simulink model "main_adaptive"  (R2021b)
settings: Solver=ode45  StartTime=0.0  StopTime=80  FixedStep=0.1  RelTol=1e-4
libraries: slpidlib x6
(part 2 of 2)

== matlab function main_adaptive/Subsystem3/u3 sign 2 ==
  data: y_t input; y_t_1 input; u2_sign output; u2_dis input; u2_dis_t_1 input
function u2_sign  = u2_sing(y_t,y_t_1,u2_dis,u2_dis_t_1)
if (u2_dis-u2_dis_t_1)==0
    u2_sign=0;
else
u2_sign=sign( (y_t-y_t_1)/(u2_dis-u2_dis_t_1) );
end

== matlab function main_adaptive/u1 whit /MATLAB Function ==
  data: dz input; ddz output; phi input; theta input; u1 input; ms input; g input; k3 input
function ddz = zstate(dz,phi,theta,u1,ms,g,k3)

ddz = -g + (cos(theta)*cos(phi))/ms*u1 + (-k3*dz/ms);

end

== matlab function main_adaptive/Subsystem1/MATLAB Function1 ==
  data: dpsi input; ddpsi output; u4 input; c input; Iz input; k6 input
function ddpsi = psi_state(dpsi,u4,c,Iz,k6)

ddpsi = 0 + c/Iz*u4 + (-k6/Iz*dpsi);

end

== matlab function main_adaptive/u1 whit /sliding surface for z ==
  data: wz input; s_z output; z input; zd input; dz input; dzd input
function s_z = sliding_sur_z(wz,z,zd,dz,dzd)

s_z=wz*(zd-z)+(dzd-dz);

end

== matlab function main_adaptive/u1 whit /u1 ==
  data: dz input; phi input; u1 output; theta input; dzd input; ddzd input; ms input; g input; wz input; epsilonz input; s_z input; u1_dis output
function [u1,u1_dis] = u1_function(dz,phi,theta,dzd,ddzd,ms,g,wz,epsilonz,s_z)

u1_dis = ms/(cos(theta)*cos(phi))*(epsilonz*tanh(s_z));
u1 = ms/(cos(theta)*cos(phi))*(wz*(dzd - dz) + ddzd + g) + ms/(cos(theta)*cos(phi))*(epsilonz*tanh(s_z));
end

== matlab function main_adaptive/u1 whit /u1 sign ==
  data: z_t input; z_t_1 input; u1_sign output; u1_dis input; u1_dis_t_1 input
function u1_sign  = u1_sing(z_t,z_t_1,u1_dis,u1_dis_t_1)
if (u1_dis-u1_dis_t_1) == 0
    u1_sign=0;
else
    u1_sign=sign( (z_t-z_t_1)/(u1_dis-u1_dis_t_1) );
end
end
